simulink model "Execution_servo_tangage_1_v2_corrige"  (R2013a)
settings: Solver=FixedStepDiscrete  StartTime=0.0  StopTime=inf  RelTol=1e-3
libraries: arduino_io_lib x5
settings Model: Creator=Francois  LastModifiedBy=Propriétaire
settings DataIOCC: SignalLoggingSaveFormat=ModelDataLogs
settings OptimizationCC: ExpressionDepthLimit=2147483647
settings DebuggingCC: FcnCallInpInsideContextMsg=EnableAllAsWarning

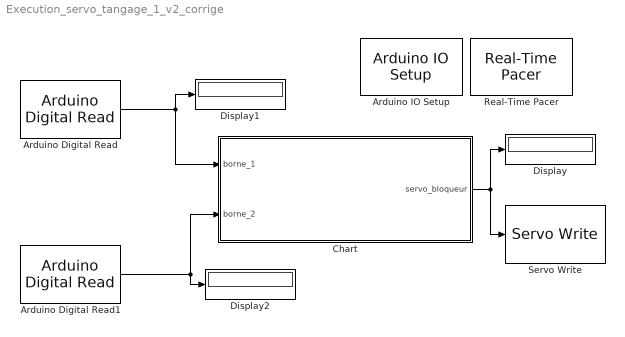
== system Execution_servo_tangage_1_v2_corrige ==
  Arduino Digital Read : arduino_io_lib/Arduino Digital Read  arduinoVar=Temporary arduino variable: Arduino1  arduinoPin=2  T=0.2
  Arduino Digital Read1 : arduino_io_lib/Arduino Digital Read  arduinoVar=Temporary arduino variable: Arduino1  arduinoPin=4  T=0.2
  Arduino IO Setup : arduino_io_lib/Arduino IO Setup  Priority=3  arduinoVar=Temporary arduino variable: Arduino1  workspaceVarName=a  comPort=COM49
  Chart : Stateflow chart  TreatAsAtomicUnit=on
  Display : Display
  Display1 : Display
  Display2 : Display
  Real-Time Pacer : arduino_io_lib/Real-Time Pacer  simTimePerRealTime=1
  Servo Write : arduino_io_lib/Servo Write  arduinoVar=Temporary arduino variable: Arduino1  pinNum=3  T=0.2
  wires:
  Arduino Digital Read/1 -> Display1/1, Chart/1(borne_1)
  Arduino Digital Read1/1 -> Display2/1, Chart/2(borne_2)
  Chart/1(servo_bloqueur) -> Display/1, Servo Write/1

== stateflow chart Execution_servo_tangage_1_v2_corrige/Chart ==
  state tangage_bloque
    entry : servo_bloqueur = 45;
  state tangage_libre
    entry : servo_bloqueur = 135;
  state tangage_limite
    entry : servo_bloqueur = 90;
  (default) -> (junction 24)
  (junction 24) -> tangage_libre [order 3] : [borne_1==1 && borne_2==0]
  (junction 24) -> tangage_bloque [order 1] : [borne_1==1 && borne_2==1]
  (junction 24) -> tangage_limite [order 2] : [borne_1==0 && borne_2==1]
  tangage_libre -> tangage_limite : [! borne_1]
  tangage_bloque -> tangage_limite : [borne_1 == 0 && borne_2 == 1]
  tangage_limite -> tangage_libre [order 2] : [borne_1 && !borne_2]
  tangage_limite -> tangage_bloque [order 1] : [borne_1 == 1 && borne_2 == 1]
  data: borne_1 input; borne_2 input; servo_bloqueur output double
